simulink model "acrobot_simulation_v8"  (R2018b)
settings: Solver=ode8  StartTime=0.0  StopTime=12  FixedStep=0.01  RelTol=1e-3
model workspace (MAT data in the model file):
  g = 9.81
  l1 = 0.6
  l2 = 0.5
  m1 = 1
  m2 = 10
values from neighbouring files (symbols this model uses):
  As = [zeros(size(D,1))     eye(size(D,1)) ... (first row only)    [LQR_balance.m]
  Bs = [zeros(size(D,1),size(B,2)) ... (first row only)    [LQR_balance.m]
  Cs = eye(size(As,1))    [LQR_balance.m]
  Ds = zeros(size(Cs,1),size(Bs,2))    [LQR_balance.m]
  K = lqr(As,Bs,Q,R)    [LQR_balance.m]
undefined symbols (not defined in the file or in its folder): param
libraries: simulink x1
settings Model: Creator=oguzhan  LastModifiedBy=oguzh
settings SFSimCC: SimUseLocalCustomCode=off
settings RTWCC: RTWUseLocalCustomCode=off
settings CodeAppCC: StateflowObjectComments=on

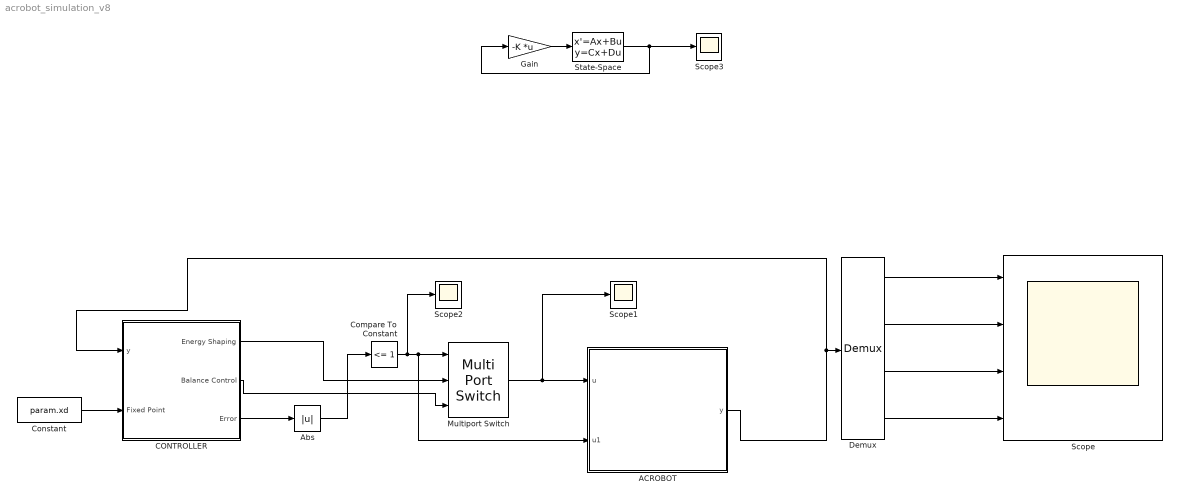
== system acrobot_simulation_v8 ==
  ACROBOT : Subsystem
      mask Display: image(imread('acrobot.png'))
  Abs : Abs
  CONTROLLER : Subsystem
  Compare To Constant : simulink/Logic and Bit Operations/Compare To Constant  relop=<=  const=1  OutDataTypeStr=boolean
  Constant : Constant  Value=param.xd
  Demux : Demux
  Gain : Gain  Gain=-K  Multiplication=Matrix(K*u) (u vector)
  Multiport Switch : MultiPortSwitch  DataPortOrder=Zero-based contiguous  Inputs=2  zeroidx=on
  Scope : Scope  NumInputPorts=4
  Scope1 : Scope
  Scope2 : Scope
  Scope3 : Scope
  State-Space : StateSpace  A=As  B=Bs  C=Cs  D=Ds  InitialCondition=pi/2
  wires:
  ACROBOT/1(y) -> CONTROLLER/1(y), Demux/1
  Constant/1 -> CONTROLLER/2(Fixed Point)
  Demux/1 -> Scope/1
  CONTROLLER/1(Energy Shaping) -> Multiport Switch/2
  CONTROLLER/2(Balance Control) -> Multiport Switch/3
  Multiport Switch/1 -> Scope1/1, ACROBOT/1(u)
  Demux/2 -> Scope/2
  Demux/3 -> Scope/3
  Demux/4 -> Scope/4
  State-Space/1 -> Gain/1, Scope3/1
  Gain/1 -> State-Space/1
  CONTROLLER/3(Error) -> Abs/1
  Compare To Constant/1 -> Scope2/1, ACROBOT/2(u1), Multiport Switch/1
  Abs/1 -> Compare To Constant/1

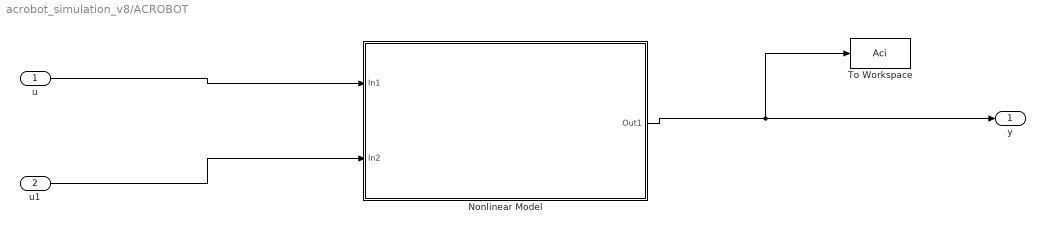
== system acrobot_simulation_v8/ACROBOT ==
  u : Inport
  u1 : Inport  Port=2
  Nonlinear Model : Subsystem
  To Workspace : ToWorkspace  VariableName=Aci  SaveFormat=Structure  SampleTime=-1
  y : Outport
  wires:
  u/1 -> Nonlinear Model/1(In1)
  Nonlinear Model/1(Out1) -> To Workspace/1, y/1
  u1/1 -> Nonlinear Model/2(In2)

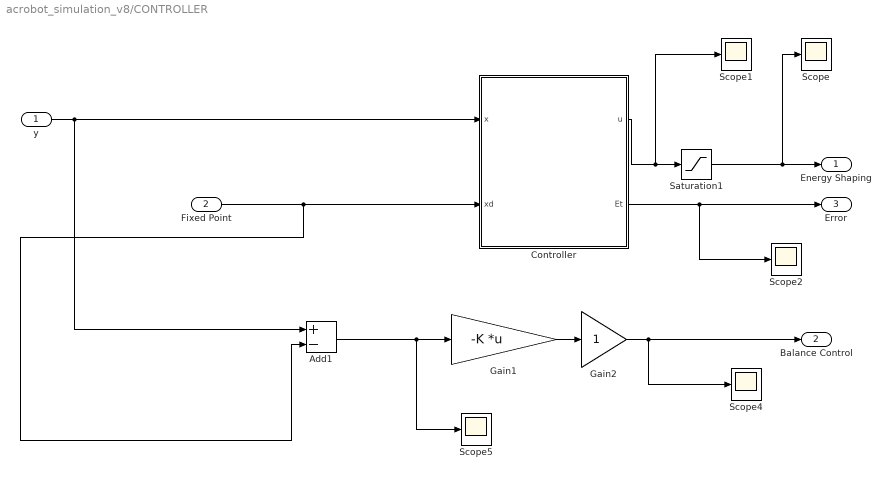
== system acrobot_simulation_v8/CONTROLLER ==
  y : Inport
  Fixed Point : Inport  Port=2
  Add1 : Sum  Inputs=+-
  Controller : MATLAB Function  TreatAsAtomicUnit=on
  Gain1 : Gain  Gain=-K  Multiplication=Matrix(K*u) (u vector)
  Gain2 : Gain
  Saturation1 : Saturate  UpperLimit=75  LowerLimit=-75
  Scope{,1..2,4..5} (5 alike) : Scope
  Energy Shaping : Outport
  Balance Control : Outport  Port=2
  Error : Outport  Port=3
  wires:
  Fixed Point/1 -> Add1/2, Controller/2(xd)
  Controller/1(u) -> Scope1/1, Saturation1/1
  Saturation1/1 -> Scope/1, Energy Shaping/1
  Gain1/1 -> Gain2/1
  Add1/1 -> Gain1/1, Scope5/1
  Gain2/1 -> Balance Control/1, Scope4/1
  y/1 -> Add1/1, Controller/1(x)
  Controller/2(Et) -> Error/1, Scope2/1

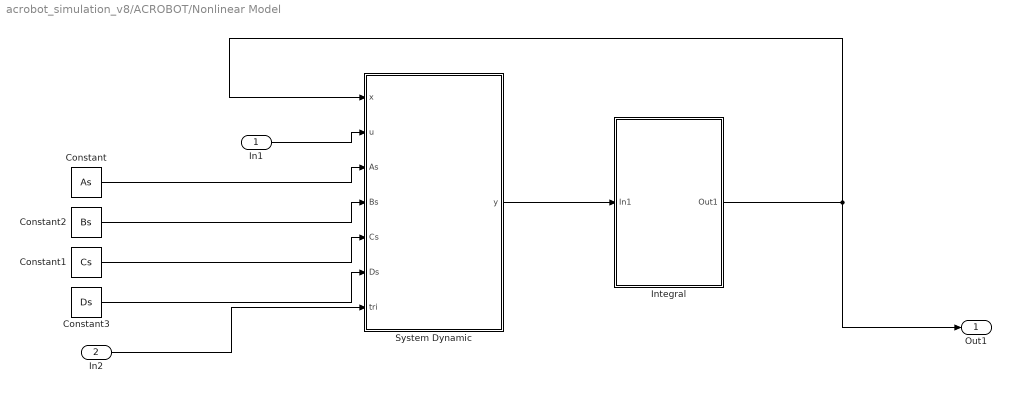
== system acrobot_simulation_v8/ACROBOT/Nonlinear Model ==
  In1 : Inport
  In2 : Inport  Port=2
  Constant : Constant  Value=As
  Constant1 : Constant  Value=Cs
  Constant2 : Constant  Value=Bs
  Constant3 : Constant  Value=Ds
  Integral : Subsystem
  System Dynamic : MATLAB Function  TreatAsAtomicUnit=on
  Out1 : Outport
  wires:
  Integral/1(Out1) -> Out1/1, System Dynamic/1(x)
  System Dynamic/1(y) -> Integral/1(In1)
  In1/1 -> System Dynamic/2(u)
  Constant/1 -> System Dynamic/3(As)
  Constant1/1 -> System Dynamic/5(Cs)
  Constant2/1 -> System Dynamic/4(Bs)
  Constant3/1 -> System Dynamic/6(Ds)
  In2/1 -> System Dynamic/7(tri)

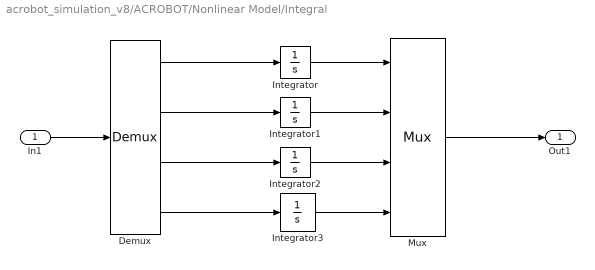
== system acrobot_simulation_v8/ACROBOT/Nonlinear Model/Integral ==
  In1 : Inport
  Demux : Demux
  Integrator : Integrator  WrapState=on  WrappedStateUpperValue=2*pi  WrappedStateLowerValue=0
  Integrator1 : Integrator  InitialCondition=pi/6  WrappedStateUpperValue=2*pi  WrappedStateLowerValue=0
  Integrator2 : Integrator
  Integrator3 : Integrator
  Mux : Mux
  Out1 : Outport
  wires:
  In1/1 -> Demux/1
  Integrator1/1 -> Mux/2
  Integrator2/1 -> Mux/3
  Demux/2 -> Integrator1/1
  Demux/3 -> Integrator2/1
  Demux/1 -> Integrator/1
  Integrator/1 -> Mux/1
  Demux/4 -> Integrator3/1
  Integrator3/1 -> Mux/4
  Mux/1 -> Out1/1

== matlab function acrobot_simulation_v8/CONTROLLER/Controller ==
  data: x input; u output; xd input; Et output
function [u,Et]= fcn(x,xd)
%% Parameters
m1=1.6 ; %Mass of lover Pendulum
m2=2 ;%Mass of upper Pendulum
l1=0.42 ; %Lower Pendulum Length
l2=0.3 ;%Upper Pendulum Length
g=9.81 ;%Gravity

xd=[pi
    0
    0
    0]; %% fixed point
%% measurement Decompozition


n=length(x);

q=x(1:n/2);
dq=x(n/2+1:n);
%% Position Equations
p1=l1*[sin(q(1))
       cos(q(1))];  
   
dp1=l1*dq(1)*[cos(q(1))
             -sin(q(1))];
         
         
p2=p1+l2*[sin(q(1)+q(2))
          cos(q(1)+q(2))];
   
dp2=dp1 + l2*(dq(1)+dq(2))*[cos(q(1)+q(2))
                           -sin(q(1)+q(2))]; 
                       
dp=[dp1
    dp2];

%% Energy Equation
qd=xd;
Ek=(1/2)*(m1*(dp1'*dp1)+m2*(dp2'*dp2)); %Kinetic Energy

Ep= - m1*g*l1*cos(q(1)) - m2*g*(l1*cos(q(1))+l2*cos(q(1)+q(2))); %Potantial Energy


E=Ek+Ep; %Total Energy


Ed=-m1*g*l1*cos(qd(1)) - m2*g*(l1*cos(qd(1))+l2*cos(qd(1)+qd(2))); % Desired Energy


Et=E-Ed; % Energy Level Error

%% Controller Output
u=-((dq(2)+1.51)*Et);

== matlab function acrobot_simulation_v8/ACROBOT/Nonlinear Model/System Dynamic ==
  data: y output; x input; u input; As input; Bs input; Cs input; Ds input; tri input
function y  = Acrobot(x,u,As,Bs,Cs,Ds,tri)
y=zeros(4,1);
%% parameters
m1=1.6 ; %Mass of lover Pendulum
m2=2 ;%Mass of upper Pendulum
l1=0.42 ; %Lower Pendulum Length
l2=0.3 ;%Upper Pendulum Length
g=9.81 ;%Gravity

xd=[pi
    0
    0
    0]; %% fixed point

q=zeros(2,1);
dq=zeros(2,1);

q=x(1:2);
dq=x(3:4);

%% model
D=zeros(2,2);
C=zeros(2,2);
G=zeros(2,1);
B=zeros(2,1);


D(1,1)=(m1+m2)*l1^2+m2*l2^2+m2*l1*l2*cos(q(2));
D(1,2)=m2*l2^2+m2*l1*l2*cos(q(2));
D(2,1)=D(1,2);
D(2,2)=m2*l2^2;


C(1,1)=0;
C(1,2)=-m2*l1*l2*(dq(1)+dq(2))*sin(q(2));
C(2,1)=-m2*l1*l2*(dq(2))*sin(q(2));
C(2,2)=m2*l1*l2*(dq(1)+dq(2))*sin(q(2));


G(1)=(m1+m2)*l1*sin(q(1))+m2*l2*sin(q(1)+q(2));
G(2)=m2*l2*sin(q(1)+q(2));

G=g*G;


B(1)=0;
B(2)=1;

% 
if tri==1
% y=zeros(4,1);
% y=As*(x-xd)+Bs*u %ul=-K*(x-xd);
 

 %% nonlinear model   
% Dqq+Cdq+G=Bu





DC= -(D^-1)*C;

DG= -(D^-1)*G;

DB= D^-1*B;

fx=zeros(4,1);

fx(1)=dq(1);
fx(2)=dq(2);
fx(3)=DC(1,:)*dq+DG(1);
fx(4)=DC(2,:)*dq+DG(2);


gx=[zeros(size(DB,1),1)
    DB];
y=fx+gx*u;


elseif tri==0
  %% partial feedback linearized model  

h1=C(1,1)+C(1,2);
h2=C(2,1)+C(2,2);

phi1=G(1);
phi2=G(2);



fx=zeros(4,1);

fx(1)=dq(1);
fx(2)=dq(2);
fx(3)=-D(1,1)^(-1)*(h1+phi1);
fx(4)=0;

k=0.17;
kp=4.5;  %angular displacement gain
kd=1;    %angular velocity gain 


U=k*u-kp*q(2)-kd*dq(2); % designed controller

gx=[ 0
     0
    -D(1,1)^(-1)*D(1,2)*U
     U];

% y=zeros(4,1)
y=fx+gx;
end
